simulink model "part_2"  (R2017b)
settings: Solver=VariableStepAuto  StartTime=0.0  StopTime=8  MaxStep=0.001  RelTol=1e-3
settings Model: Creator=drone  LastModifiedBy=drone

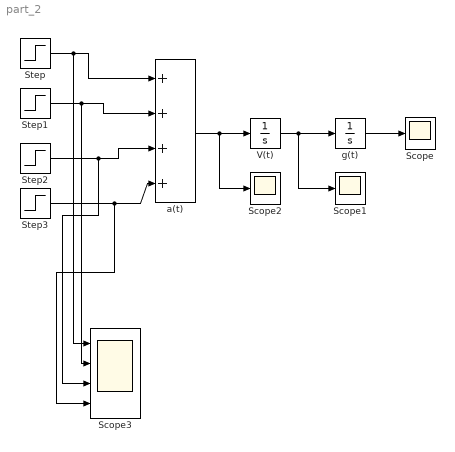
== system part_2 ==
  Scope : Scope
  Scope1 : Scope
  Scope2 : Scope
  Scope3 : Scope  NumInputPorts=4
  Step : Step  Time=0.5  Before=4  After=0  SampleTime=0
  Step1 : Step  Time=5  After=-4  SampleTime=0
  Step2 : Step  Time=5.5  Before=-4  After=0  SampleTime=0
  Step3 : Step  Time=6  Before=4  After=4  SampleTime=0
  V(t) : Integrator
  a(t) : Sum  Inputs=++++
  g(t) : Integrator
  wires:
  Step/1 -> Scope3/1, a(t)/1
  a(t)/1 -> Scope2/1, V(t)/1
  V(t)/1 -> Scope1/1, g(t)/1
  g(t)/1 -> Scope/1
  Step1/1 -> Scope3/2, a(t)/2
  Step2/1 -> Scope3/3, a(t)/3
  Step3/1 -> a(t)/4, Scope3/4
